simulink model "Prescan_Carsim_0118_cs"  (R2019b)
settings: Solver=ode5  StartTime=0.0  StopTime=inf  FixedStep=1/1000  RelTol=1e-3
PreLoadFcn:
  | mbxruntime.callbacks.PreLoadFcn(bdroot);
PostLoadFcn:
  | mbxruntime.callbacks.PostLoadFcn(bdroot);
InitFcn:
  | mbxruntime.callbacks.InitFcn(bdroot);
  | Initialization_Func;
  | 
  | % load the InputBus data.
  | load osqpcecInputBus.mat;
StartFcn:
  | mbxruntime.callbacks.StartFcn(bdroot);
  | current_sys=gcs;
  | speedblock=Simulink.findBlocks(current_sys,'Name','speed_kmh_Gain');
  | h1=add_exec_event_listener(speedblock,'PostOutputs',@SpeedVisulization);
  | outblock=Simulink.findBlocks(current_sys,'Name','trajectorycurveoutput_Gain');
  | CurveTrajectoryListenerHandle=add_exec_event_listener(outblock,'PostOutputs',@TrajectoryCurve_CallBack);
  | lanedatablock=Simulink.findBlocks(current_sys,'Name','LaneData_Gain');
  | CurveLaneListenerHandle=add_exec_event_listener(lanedatablock,'PostOutputs',@CurveLane_CallBack);
StopFcn:
  | mbxruntime.callbacks.StopFcn(bdroot);
model workspace: external: MAT-File .\Prescan_Carsim_0118_cs_hws.mat (data not in the file)
values from neighbouring files (symbols this model uses):
  g = 9.8    [Initialization_Func.m]
  InitialPlanningParameter = [0,0,1,0,2,2,2,40,60]'    [Initialization_Func.m]
  Kf = 20000    [Initialization_Func.m]
  Kr = 20000    [Initialization_Func.m]
  Lr = 1.644    [Initialization_Func.m]
  M = 1275    [Initialization_Func.m]
  nG = 24    [Initialization_Func.m]
  V = 60/3.6    (= 16.6666666667)    [Initialization_Func.m]
  VehicleBaseLength = Lf+Lr    (= 2.66)    [Initialization_Func.m]
undefined symbols (not defined in the file or in its folder): AAx, AAy, AAz, AVx, AVy, AVz, Ax, Ay, Az, canChannel, DiscIntNeverNeededParam, InitialDPMPDF_Comfort, InitialDPMPDF_Efficiency, InitialDPMPDF_Safety, InitialPDF_DEM, mbxruntime, NormalisedTrajectoryIndicator_Pool, Parameter_Indicator_LookUpTable, Prescan_Carsim_1230_cs_0658e9ca1334a8be, Prescan_Carsim_1230_cs_08c5eb9a1bd7376a, Prescan_Carsim_1230_cs_6cfd759b89b9fc85, Prescan_Carsim_1230_cs_9435cc1cceb5050d, Prescan_Carsim_1230_cs_ac716d34d49f74ab, Prescan_Carsim_1230_cs_be02757d7f212dd5, Rational_Coefficient_Learning, SteeringWheel, TrajectoryIndicatorRange, Vx, Vy, Vz, WheelL0, WheelL1, WheelR0, WheelR1
libraries: canmsglib x11, dsparch4 x6, canlib x3, PreScanSimulinkLibrary x3, Solver_SF x1, autolibshared x1
(part 8 of 8)

== matlab function Prescan_Carsim_0118_cs/BMW_X5_SUV_1/trajectory planning/Specific Curve Trajectory Planning/Trajectory Planning For Curve under beginning-global/Subsystem/Path Planning_OSQP Transformation ==
  data: RoadLaneBorder_ForPlan input size=[1000 4]; mode_Length output Bus: osqpcecInput; mode2_Curveture output Bus: osqpcecInput; mode4_HeadingError output Bus: osqpcecInput
function [mode_Length,mode2_Curveture,mode4_HeadingError]= PathPlanningMode(RoadLaneBorder_ForPlan)
% alpha_path_length: the solution of the shortest path
% alpha_curvature:the solution of the minimum curvature
% alpha_centering:the solution of the centering 
% alpha_heading_error:the solution of the minimum heading error
Num_point=size(RoadLaneBorder_ForPlan,1);
Xl=RoadLaneBorder_ForPlan(:,1);
Yl=RoadLaneBorder_ForPlan(:,2);
Xr=RoadLaneBorder_ForPlan(:,3);
Yr=RoadLaneBorder_ForPlan(:,4);

lb = 0.2*ones(size(Xr,1),1);
ub = 0.80*ones(size(Xr,1),1);
lb(1:3) = Init_pos;
ub(1:3)=Init_pos;
lb(end-2:end) = Init_pos;
ub(end-2:end)=Init_pos;
%     lb(end) = 0.5;
%     ub(end) = 0.5;

% Quadratic programming
delta_X = Xl - Xr;% (n+1)*1
delta_Y = Yl - Yr;
% objective function of minimum distance
H_dist = diag(2*delta_X.*delta_X)+diag(-delta_X(1:end-1).*delta_X(2:end),-1)...
    +diag(-delta_X(1:end-1).*delta_X(2:end),1)+diag(2*delta_Y.*delta_Y)...
    +diag(-delta_Y(1:end-1).*delta_Y(2:end),-1)...
    +diag(-delta_Y(1:end-1).*delta_Y(2:end),1);
H_dist(1, 1) = delta_X(1).*delta_X(1)+delta_Y(1).*delta_Y(1);
H_dist(end, end) = delta_X(end).*delta_X(end)+delta_Y(end).*delta_Y(end);
B_dist_con = diag(ones(1,Num_point)*4)...
    +diag(ones(1,Num_point-1)*-2,-1)+diag(ones(1,Num_point-1)*-2,1);
B_dist_con(1,1) = 2; B_dist_con(end,end) = 2;
B_dist = diag(delta_X)*B_dist_con*Xr + diag(delta_Y)*B_dist_con*Yr;
H_dist_qp = H_dist * 2;

% objective function of minimum curvature
M = diag(ones(1,Num_point)*4)+diag(ones(1,Num_point-1),-1)+diag(ones(1,Num_point-1),1);
M(1,1) = 2; 
M(end,end) = 2;
N = diag(ones(1,Num_point-1)*-1,-1)+diag(ones(1,Num_point-1),1);
N(1,1) = -1; N(end,end) = 1;
O = diag(ones(1,Num_point)*-1)+diag(ones(1,Num_point-1),1);
O(end,:) = [];
P=diag(ones(1,Num_point)*2)+diag(ones(1,Num_point-1),1);
P(end,:) = [];
D = 6 * (O - P* pinv(M) * N);
H_tao=diag(delta_X)'*(D'*D)*diag(delta_X) + diag(delta_Y)'*(D'*D)*diag(delta_Y);
B_tao=(2*Xr'*(D'*D)*diag(delta_X) + 2*Yr'*(D'*D)*diag(delta_Y))';
H_tao_qp = H_tao*2;

% objective function of minimum heading error
H_P = diag(2*ones(1,Num_point))+diag(-1*ones(1,Num_point-1),1)+diag(-1*ones(1,Num_point-1),-1);%(n+1)*(n+1)
H_P(1,1)=1;
H_P(end,end)=1;
B_HeadingError = zeros(size(Xr,1),1);
H_head_qp = 2*H_P;

% QP parameters
EyeM = eye(Num_point);
mode_Length = osqpcecPara(H_dist_qp,B_dist, EyeM, lb, ub);
mode2_Curveture = osqpcecPara(H_tao_qp,B_tao, EyeM, lb, ub);
mode4_HeadingError = osqpcecPara(H_head_qp,B_HeadingError, EyeM, lb, ub);
end

% OSQP parameter calculation
function para = osqpcecPara(P, q, A, L, u)
maxLenM = 10000;
maxLenV = 100;
para = struct('m',int32(0), 'n',int32(0), 'P_nnz',int32(0), 'P_x',zeros(maxLenM, 1, 'double'),...
    'P_i',zeros(maxLenM, 1, 'int32'), 'P_p',zeros(maxLenV, 1, 'int32'), 'q',zeros(maxLenV, 1, 'double'),...
    'A_nnz',int32(0), 'A_x',zeros(maxLenM, 1, 'double'), 'A_i',zeros(maxLenM, 1, 'int32'),...
    'A_p',zeros(maxLenV, 1, 'int32'), 'l',zeros(maxLenV, 1, 'double'), 'u',zeros(maxLenV, 1, 'double'));
para.m = int32(size(P,1));
para.n = int32(size(A,1));
[P_x, P_i, P_p, P_nnz] = Mat2CSC(triu(P)); % UTM format is needed for P first. 1215
para.P_nnz = P_nnz;
para.P_x(1:P_nnz) = P_x;
para.P_i(1:P_nnz) = P_i;
para.P_p(1:para.m+1) = P_p;
para.q(1:para.m) = q;
[A_x, A_i, A_p, A_nnz] = Mat2CSC(A);
para.A_nnz = A_nnz;
para.A_x(1:A_nnz) = A_x;
para.A_i(1:A_nnz) = A_i;
para.A_p(1:para.m+1) = A_p;
para.l(1:para.n) = L;
para.u(1:para.n) = u;
end

% Converting a matrix to CSC formart
function [v, r, c1, nnz] = Mat2CSC(A)
[r, c, v] = find(sparse(A));
c1 = zeros(size(A,2)+1, 1, 'int32');
nnz = int32(length(r));
for i = 1 : nnz; c1(c(i)+1) = c1(c(i)+1) + 1; end
c1 = cumsum(int32(c1));
r = int32(r-1);
end

== matlab function Prescan_Carsim_0118_cs/BMW_X5_SUV_1/trajectory planning/Specific Curve Trajectory Planning/Trajectory Planning For Curve under beginning-global/Subsystem/Path merging and Speed OSQP Transformation ==
  data: alpha_path_length input; pathPolyX output; alpha_curvature input; RoadLaneBorder_ForPlan input size=[1000 4]; pathPolyY output; pathInterpX output; pathInterpY output; Speedlp output Bus: osqpcecInput; Parameter_PathPlan input size=[9 1]
function [pathPolyX, pathPolyY, pathInterpX, pathInterpY, Speedlp]=PathPlan(alpha_path_length,alpha_curvature,RoadLaneBorder_ForPlan,Parameter_PathPlan)


Num_point=size(RoadLaneBorder_ForPlan,1);
Xl=RoadLaneBorder_ForPlan(:,1);
Yl=RoadLaneBorder_ForPlan(:,2);
Xr=RoadLaneBorder_ForPlan(:,3);
Yr=RoadLaneBorder_ForPlan(:,4);

% Hyper parameters
ptInterp = 5;        % path interpolation density
ptCurv = 10;         % smoothing window of curvature calculation
miu = 0.8;           % supposed friction coefficient, -
gravity = 9.8;       % gravity acceleration, m-s^-2

% Path merging
alpha1 = alpha_path_length(1:Num_point);
alpha2 = alpha_curvature(1:Num_point);
alpha3 = repmat(0.5, Num_point, 1);
alpha4 = alpha40(1:Num_point);
alpha = beta1 * alpha1 + beta2 * alpha2 + beta3 * alpha3...
    + (1 - beta1 - beta2 - beta3) * alpha4;
Parameter_PathPlan=[beta1, beta2,beta3, latA, accA, decA, minV0, maxV0];


%{
Parameter_PathPlan=Parameter_TrajectoryPlan(1:4,1);
if sum(Parameter_TrajectoryPlan(1:3)>1)
    Parameter_PathPlan=[0,0,1,0.5];
end    
% fixed lateral offst
alpha_fixlatoff=ones(Num_LanePlan,1)*Parameter_PathPlan(4);
sign_center=sign(Parameter_PathPlan(4)-Init_pos);
offset=0.02;
alpha_fixlatoff(1:3)=Init_pos;% consistent within the pathplanning function
alpha_fixlatoff(4:21)=pchip([1,5,14,18],[Init_pos,Init_pos+sign_center*offset,Parameter_PathPlan(4)-sign_center*offset,Parameter_PathPlan(4)],(1:18));
alpha_fixlatoff(end-2:end)=Init_pos;
% alpha_heading(4:6)=spline([1,5],[Init_pos,Parameter_PathPlan(4)],(2:4));
% alpha_heading(end-5:end-3)=spline([1,5],[Parameter_PathPlan(4),Init_pos],(2:4));
alpha_fixlatoff(end-20:end-3)=pchip([1,5,14,18],[Parameter_PathPlan(4),Parameter_PathPlan(4)-sign_center*offset,Init_pos+sign_center*offset,Init_pos],(1:18));

alpha=[alpha_path_length,alpha_curvature,alpha_fixlatoff]*Parameter_PathPlan(1:3,1);% Num_roadseg*Num_beta
% end
Path_PlanTemp(1:Num_LanePlan,1) = RightBound(:,1) + (LeftBound(:,1)-RightBound(:,1)).* alpha;
Path_PlanTemp(1:Num_LanePlan,2)= RightBound(:,2) + (LeftBound(:,2)-RightBound(:,2)).* alpha;
Path_Plan_Local=Path_PlanTemp;
PlanPathDataLength_Curve=Num_LanePlan;

% Convert the Local path to global path
PathPlan_Global=Transfer2Global(Path_Plan_Local,VehicleState_Beginning);
% HeadingAngle_Beginning_rad=VehicleState_Beginning(3);
% Rotation_Beginning=[cos(HeadingAngle_Beginning_rad),-sin(HeadingAngle_Beginning_rad); sin(HeadingAngle_Beginning_rad),cos(HeadingAngle_Beginning_rad)];
% PathPlan_Beginning_temp=Path_Plan_Local(:,1:2)*Rotation_Beginning';
% PathPlan_Global=[PathPlan_Beginning_temp(:,1)+VehicleState_Beginning(1),...
%     PathPlan_Beginning_temp(:,2)+VehicleState_Beginning(2)];
  
% Speed_Profile planning
% step 1, Calculate the curvature of the path
Curvature=Curvature_cal(Path_Plan_Local(1:Num_LanePlan,1),Path_Plan_Local(1:Num_LanePlan,2));
Curvature(1:10)=0;
Curvature(end-9:end)=0;

Parameter_SpeedPlan=Parameter_TrajectoryPlan(5:end,1);
% The speed plan parameters
LatAcceleration_Limit=Parameter_SpeedPlan(1);% m/s2
LongidAcceleration_Limit=Parameter_SpeedPlan(2);% m/s2
LongidDeceleration_Limit=Parameter_SpeedPlan(3);% m/s2
Velocity_LowerBound=Parameter_SpeedPlan(4)/3.6;% m/s
Velocity_UpperBound=Parameter_SpeedPlan(5)/3.6;% m/s
% Begin speed plan
Speed_Planned_kmh=zeros(1000,1);

SpeedProfile_Temp=Speedprofile(Num_LanePlan,Curvature,LatAcceleration_Limit,LongidAcceleration_Limit,...
LongidDeceleration_Limit,Velocity_LowerBound,Velocity_UpperBound);% the speedProfile is a 1000*1 data array
% smooth the speed
% span = 5;
% SpeedProfile_Temp=smooth_solver(SpeedProfile_Temp,span);
Speed_Planned_kmh(1:Num_LanePlan,1)=SpeedProfile_Temp*3.6;% km/h
%}



% Matrixs needed basically
A = diag(ones(1,Num_point)*4)+diag(ones(1,Num_point-1),-1)+diag(ones(1,Num_point-1),1);
A(1,1) = 2; A(end,end) = 2;
B = diag(ones(1,Num_point-1)*-1,-1)+diag(ones(1,Num_point-1),1);
B(1,1) = -1; B(end,end) = 1;
G = 3 * A \ B;
delta_X = Xl-Xr;% (n+1)*1
delta_Y = Yl-Yr;% (n+1)*1
XtsTem = Xr + delta_X .* alpha;
YtsTem = Yr + delta_Y .* alpha;
DX = G * XtsTem;
DY = G * YtsTem;

% Path polygon parameters
pathPolyX = zeros(size(XtsTem,1)-1,4);
pathPolyY = zeros(size(YtsTem,1)-1,4);
for i = 1:size(XtsTem,1)-1
    pathPolyX(i,4) = XtsTem(i);
    pathPolyX(i,3) = DX(i);
    pathPolyX(i,2) = 3*(XtsTem(i+1)-XtsTem(i))-(2*DX(i)+DX(i+1));
    pathPolyX(i,1) = 2*(XtsTem(i)-XtsTem(i+1))+DX(i)+DX(i+1);
    pathPolyY(i,4) = YtsTem(i);
    pathPolyY(i,3) = DY(i);
    pathPolyY(i,2) = 3*(YtsTem(i+1)-YtsTem(i))-(2*DY(i)+DY(i+1));
    pathPolyY(i,1) = 2*(YtsTem(i)-YtsTem(i+1))+DY(i)+DY(i+1);
end
    
% Path interpreted points
ptNum = ptInterp*(size(XtsTem,1)-1)+1;
pathSeq = 1:ptInterp:ptNum;
pathInterpX = zeros(ptNum, 1);
pathInterpY = zeros(ptNum, 1);
for i = 1:size(XtsTem,1)-1
    if i == 1; ptStart = 1; else; ptStart = pathSeq(i)+1; end
    ptEnd = pathSeq(i+1);
    ptRange = (ptStart-pathSeq(i):ptEnd-pathSeq(i))/(pathSeq(i+1)-pathSeq(i));
    pathInterpX(ptStart:ptEnd) = polyval(pathPolyX(i,:), ptRange);
    pathInterpY(ptStart:ptEnd) = polyval(pathPolyY(i,:), ptRange);
end

% Curvature of the path
curv = pathCurv(pathInterpX, pathInterpY, pathSeq, ptCurv);

% Speed planning parameters
maxV2 = sqrt(1.0./curv.*latA);      % side acceleration limit
maxV3 = maxV0.*ones(size(curv,1),1);% origin max speed limit
maxV4 = sqrt(miu*gravity./curv);        % slipping limit
maxV = min(min(maxV2,maxV3),maxV4);       % mixed max speed limit
minV = minV0.*ones(size(curv,1),1);% min speed limit
Plp = 2.0*eye(size(curv,1));           % to maximize speed under these limits
qlp = -2.0*maxV;
Alp = [G.*2;eye(size(curv,1));];                   % acceleration limit also considered
llp = [decA*ones(size(curv,1),1); minV];
ulp = [accA*ones(size(curv,1),1); maxV];
Speedlp = osqpcecPara(Plp, qlp, Alp, llp, ulp);
% paralp = 0;
end

% Curvature calculation 
function crv1 = pathCurv(x0, y0, seg, smt)
crv1 = zeros(length(seg),1);
for ii = 1:length(seg)
    jj = seg(ii)-floor(smt/2);
    if jj<1
        jj = 1;
    elseif jj>length(x0)-smt+1
        jj = length(x0)-smt+1;
    end
    x = x0(jj:jj+smt-1,1);
    y = y0(jj:jj+smt-1,1);
    A=[x,y,ones(length(x),1)];
    B=-1*(x.^2+y.^2);
    coef=A\B; % Circle fitting
    crv1(ii)= 2/sqrt(coef(1)^2+coef(2)^2-4*coef(3));
end
end

% OSQP parameter calculation
function para = osqpcecPara(P, q, A, L, u)
maxLenM = 10000;
maxLenV = 100;
para = struct('m',int32(0), 'n',int32(0), 'P_nnz',int32(0), 'P_x',zeros(maxLenM, 1, 'double'),...
    'P_i',zeros(maxLenM, 1, 'int32'), 'P_p',zeros(maxLenV, 1, 'int32'), 'q',zeros(maxLenV, 1, 'double'),...
    'A_nnz',int32(0), 'A_x',zeros(maxLenM, 1, 'double'), 'A_i',zeros(maxLenM, 1, 'int32'),...
    'A_p',zeros(maxLenV, 1, 'int32'), 'l',zeros(maxLenV, 1, 'double'), 'u',zeros(maxLenV, 1, 'double'));
para.m = int32(size(P,1));
para.n = int32(size(A,1));
[P_x, P_i, P_p, P_nnz] = Mat2CSC(triu(P)); % UTM format is needed for P first. 1215
para.P_nnz = P_nnz;
para.P_x(1:P_nnz) = P_x;
para.P_i(1:P_nnz) = P_i;
para.P_p(1:para.m+1) = P_p;
para.q(1:para.m) = q;
[A_x, A_i, A_p, A_nnz] = Mat2CSC(A);
para.A_nnz = A_nnz;
para.A_x(1:A_nnz) = A_x;
para.A_i(1:A_nnz) = A_i;
para.A_p(1:para.m+1) = A_p;
para.l(1:para.n) = L;
para.u(1:para.n) = u;
end

% Converting a matrix to CSC formart
function [v, r, c1, nnz] = Mat2CSC(A)
[r, c, v] = find(sparse(A));
c1 = zeros(size(A,2)+1, 1, 'int32');
nnz = int32(length(r));
for i = 1 : nnz; c1(c(i)+1) = c1(c(i)+1) + 1; end
c1 = cumsum(int32(c1));
r = int32(r-1);
end

== matlab function Prescan_Carsim_0118_cs/BMW_X5_SUV_1/trajectory planning/Specific Curve Trajectory Planning/Trajectory Planning For Curve under beginning-global/Subsystem/MATLAB Function ==
  data: RoadLane_Plan input; RoadLaneBorder_ForPlan output size=[1000 4]; VehicleWidth input; LaneWidth input; Num_LanePlan output
function [RoadLaneBorder_ForPlan,Num_LanePlan]= Path_OSQP(RoadLane_Plan,VehicleWidth,LaneWidth)
%Road Lane
Num_LanePlan=size(RoadLane_Plan,1);
LeftLane_Plan=RoadLane_Plan(:,1:2);
RightLane_Plan=RoadLane_Plan(:,3:4);
X_LaneLeftToRight=RightLane_Plan(:,1)-LeftLane_Plan(:,1);
Y_LaneLeftToRight=RightLane_Plan(:,2)-LeftLane_Plan(:,2);
Vec_LeftToRight=[X_LaneLeftToRight,Y_LaneLeftToRight];
LaneWidth_Estimated=sqrt(sum(Vec_LeftToRight.*Vec_LeftToRight,2));
UnitVec_LeftRight=Vec_LeftToRight./[LaneWidth_Estimated,LaneWidth_Estimated];
LaneCenter=zeros(Num_LanePlan,2);
LaneCenter(:,1)=0.5*(LeftLane_Plan(:,1)+RightLane_Plan(:,1));
LaneCenter(:,2)=0.5*(LeftLane_Plan(:,2)+RightLane_Plan(:,2));
LeftBound=LaneCenter-(LaneWidth-VehicleWidth)*0.5*UnitVec_LeftRight; % The Path Bound Should consider the Vehicle Width
RightBound=LaneCenter+(LaneWidth-VehicleWidth)*0.5*UnitVec_LeftRight;
RoadLaneBorder_ForPlan=[LeftBound,RightBound];
end
